simulink model "ResonantConverter_GaN"  (R2016a)
settings: Solver=VariableStepAuto  StartTime=0.0  StopTime=0.1  RelTol=1e-3
libraries: powerlib x18, powerlib_meascontrol x1
settings Model: Creator=syf  LastModifiedBy=syf

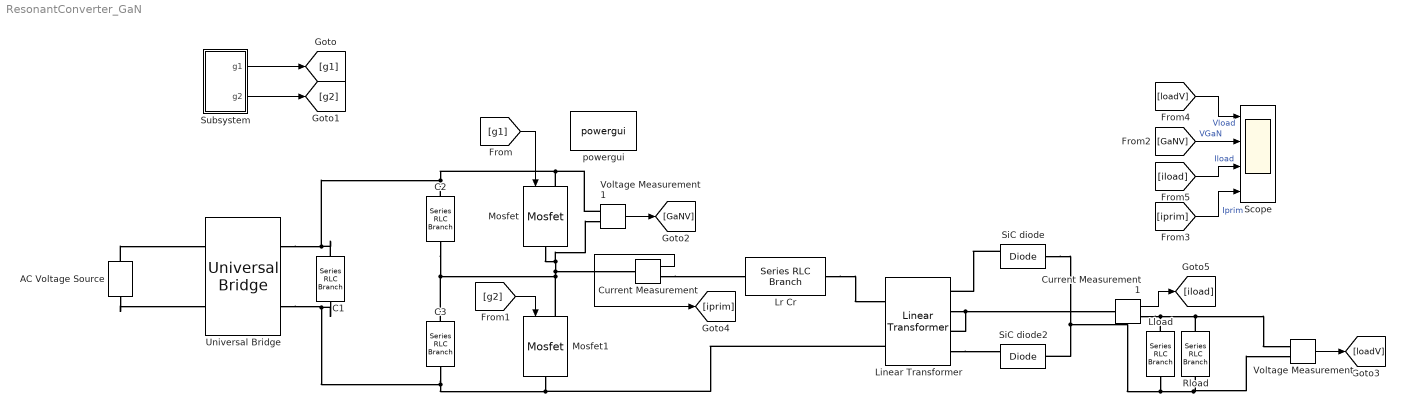
== system ResonantConverter_GaN ==
  AC Voltage Source : powerlib/Electrical Sources/AC Voltage Source  Amplitude=230*sqrt(6)  Phase=0  Frequency=60  SampleTime=0  Measurements=None  BusType=swing  Pref=10e3  Qref=0  Qmin=-inf  Qmax=+inf
  C1 : powerlib/Elements/Series RLC Branch  LConnTagsString=__new0  RConnTagsString=__new0  BranchType=C  Resistance=1  Inductance=1e-3  SetiL0=off  InitialCurrent=0  Capacitance=1e-6  Setx0=off  InitialVoltage=0  Measurements=None
  C2 : powerlib/Elements/Series RLC Branch  LConnTagsString=__new0  RConnTagsString=__new0  BranchType=C  Resistance=1  Inductance=1e-3  SetiL0=off  InitialCurrent=0  Capacitance=1e-6  Setx0=off  InitialVoltage=0  Measurements=None
  C3 : powerlib/Elements/Series RLC Branch  LConnTagsString=__new0  RConnTagsString=__new0  BranchType=C  Resistance=1  Inductance=1e-3  SetiL0=off  InitialCurrent=0  Capacitance=1e-6  Setx0=off  InitialVoltage=0  Measurements=None
  Current Measurement : powerlib/Measurements/Current Measurement  PhasorSimulation=off  OutputType=Complex  PSBequivalent=0
  Current Measurement1 : powerlib/Measurements/Current Measurement  PhasorSimulation=off  OutputType=Complex  PSBequivalent=0
  Linear Transformer : powerlib/Elements/Linear Transformer  UNITS=SI  NominalPower=[500 200e3 ]  winding1=[240 4.3218 3.2e-5]  winding2=[16 0.7938 0.014e-5]  ThreeWindings=on  winding3=[16 0.7938 0.014e-5]  RmLm=[1.0805e+06 3.2e-3]  Measurements=None  DataType=on
  Lload : powerlib/Elements/Series RLC Branch  LConnTagsString=__new0  RConnTagsString=__new0  BranchType=C  Resistance=1  Inductance=1e-3  SetiL0=off  InitialCurrent=0  Capacitance=100e-6  Setx0=off  InitialVoltage=0  Measurements=None
  Lr Cr : powerlib/Elements/Series RLC Branch  LConnTagsString=__new0  RConnTagsString=__new0  BranchType=LC  Resistance=1  Inductance=2.2e-6  SetiL0=off  InitialCurrent=0  Capacitance=22e-6  Setx0=off  InitialVoltage=0  Measurements=None
  Mosfet : powerlib/Power Electronics/Mosfet  Ron=130e-3  Lon=0  Rd=0.25  Vfd=2.2  IC=0  Rs=1e5  Cs=inf  Measurements=off
  Mosfet1 : powerlib/Power Electronics/Mosfet  Ron=130e-3  Lon=0  Rd=0.25  Vfd=2.2  IC=0  Rs=1e5  Cs=inf  Measurements=off
  Rload : powerlib/Elements/Series RLC Branch  LConnTagsString=__new0  RConnTagsString=__new0  BranchType=R  Resistance=100  Inductance=1e-3  SetiL0=off  InitialCurrent=0  Capacitance=1e-6  Setx0=off  InitialVoltage=0  Measurements=None
  Scope : Scope  NumInputPorts=4
  SiC diode : powerlib/Power Electronics/Diode  Ron=0.001  Lon=0  Vf=0.8  IC=0  UseSnubber=off  Rs=500  Cs=250e-9  Measurements=on
  SiC diode2 : powerlib/Power Electronics/Diode  Ron=0.001  Lon=0  Vf=0.8  IC=0  UseSnubber=off  Rs=500  Cs=250e-9  Measurements=on
  Subsystem : Subsystem
  Universal Bridge : powerlib/Power Electronics/Universal Bridge  Arms=2  SnubberResistance=1e5  SnubberCapacitance=inf  Device=Diodes  Ron=1e-3  Lon=0  ForwardVoltages="[  0  0  ]"  ForwardVoltage=0  GTOparameters=[ 10e-6 , 20e-6 ]  IGBTparameters=[ 1e-6 , 2e-6 ]  Measurements=None  Measurements_2=None  converterType=Rectifier
  Voltage Measurement : powerlib/Measurements/Voltage Measurement  PhasorSimulation=off  OutputType=Complex  PSBequivalent=0
  Voltage Measurement1 : powerlib/Measurements/Voltage Measurement  PhasorSimulation=off  OutputType=Complex  PSBequivalent=0
  powergui : powerlib/powergui  Priority=1  SimulationMode=Continuous  SolverType=Tustin/Backward Euler (TBE)  SampleTime=50e-6  frequency=60  SPID=on  DisableSnubberDevices=on  DisableRonSwitches=off  DisableVfSwitches=off  SwTol=0  DisplayEquations=off  Interpol=off  ExternalGateDelay=off  methode=off  Ts=10  FunctionMessages=off  echomessages=off  HookPort=off  EnableUseOfTLC=off  x0status=blocks  frequencyindice=60  Pbase=100e6  ErrMax=1e-4  Iterations=50  UnitsV=kV  UnitsW=MW  buscounter=0  RestoreLinks=warning  ResistiveCurrentMeasurement=off  Frange=[0:2:500]  Ylog=off  Xlog=on  ShowGrid=off  save=off  variable=ZData  structure=0  ZoomFFT=off  StartTime=0.0  cycles=1  DisplayStyle=1  fundamental=60  FreqAxis=off  MaxFrequency=1000  frequencyindicesteady=1  RmsSteady=1  display=off
  wires:
  [g2] -> Mosfet1/1
  [g1] -> Mosfet/1
  Voltage Measurement1/1 -> [GaNV]
  Voltage Measurement/1 -> [loadV]
  Current Measurement/1 -> [iprim]
  Current Measurement1/1 -> [iload]
  [loadV] -> Scope/1  "Vload"
  [GaNV] -> Scope/2  "VGaN"
  [iload] -> Scope/3  "Iload"
  [iprim] -> Scope/4  "Iprim"
  Subsystem/1("g1 ") -> [g1]
  Subsystem/2(g2) -> [g2]
  connections:
  C2/RConn1 -- C3/LConn1 -- Mosfet1/LConn1 -- Mosfet/RConn1 -- Voltage Measurement1/LConn2 -- Current Measurement/LConn1
  Linear Transformer/LConn2 -- Mosfet1/RConn1 -- C1/RConn1 -- Universal Bridge/RConn2 -- C3/RConn1
  Lr Cr/RConn1 -- Linear Transformer/LConn1
  Linear Transformer/RConn4 -- SiC diode2/RConn1
  SiC diode/RConn1 -- Linear Transformer/RConn1
  Linear Transformer/RConn2 -- Current Measurement1/LConn1 -- Linear Transformer/RConn3
  Lload/RConn1 -- Voltage Measurement/LConn2 -- Rload/RConn1 -- SiC diode2/LConn1 -- SiC diode/LConn1
  AC Voltage Source/RConn1 -- Universal Bridge/LConn1
  AC Voltage Source/LConn1 -- Universal Bridge/LConn2
  C2/LConn1 -- Mosfet/LConn1 -- Voltage Measurement1/LConn1 -- C1/LConn1 -- Universal Bridge/RConn1
  Current Measurement/RConn1 -- Lr Cr/LConn1
  Rload/LConn1 -- Current Measurement1/RConn1 -- Lload/LConn1 -- Voltage Measurement/LConn1

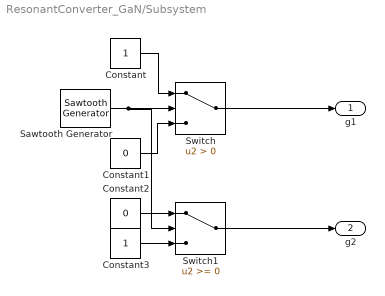
== system ResonantConverter_GaN/Subsystem ==
  Constant : Constant
  Constant1 : Constant  Value=0
  Constant2 : Constant  Value=0
  Constant3 : Constant
  Sawtooth Generator : powerlib_meascontrol/Pulse & Signal Generators/Sawtooth Generator  Freq=250e3  Phase=180  Ts=0
  Switch : Switch  Criteria=u2 > Threshold
  Switch1 : Switch
  "g1 " : Outport
  g2 : Outport  Port=2
  wires:
  Switch1/1 -> g2/1
  Sawtooth Generator/1 -> Switch1/2, Switch/2
  Switch/1 -> "g1 "/1
  Constant2/1 -> Switch1/1
  Constant1/1 -> Switch/3
  Constant3/1 -> Switch1/3
  Constant/1 -> Switch/1
